simulink subsystem "CF1_SubSystem"  (R2020b)
settings: Solver=VariableStepAuto  StartTime=0.0  StopTime=10.0  RelTol=1e-3
values from neighbouring files (symbols this model uses):
  Hz = HFE    [StateSpaceSimpleObserver.m]
  Ts = 1e-2    (= 0.01)    [balrob_params.m]
undefined symbols (not defined in the file or in its folder): DiscIntNeverNeededParam
settings Model: Creator=umberto  LastModifiedBy=umberto

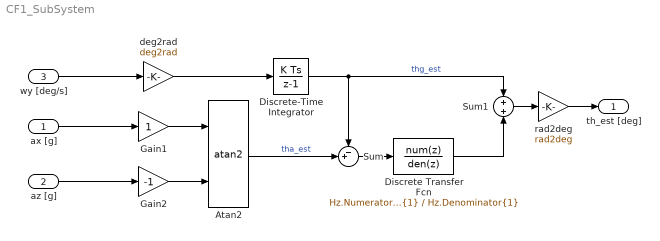
== system CF1_SubSystem ==
  ax [g] : Inport
  az [g] : Inport  Port=2
  wy [deg/s] : Inport  Port=3
  Atan2 : Trigonometry  Operator=atan2
  Discrete Transfer Fcn : DiscreteTransferFcn  Numerator=Hz.Numerator{1}  Denominator=Hz.Denominator{1}  SampleTime=Ts
  Discrete-Time Integrator : DiscreteIntegrator  SampleTime=Ts  ICPrevOutput=DiscIntNeverNeededParam  ICPrevScaledInput=DiscIntNeverNeededParam
  Gain1 : Gain
  Gain2 : Gain  Gain=-1
  Sum : Sum  Inputs=-+|
  Sum1 : Sum
  deg2rad : Gain  Gain=deg2rad
  rad2deg : Gain  Gain=rad2deg
  th_est [deg] : Outport
  wires:
  wy [deg/s]/1 -> deg2rad/1
  deg2rad/1 -> Discrete-Time Integrator/1
  ax [g]/1 -> Gain1/1
  az [g]/1 -> Gain2/1
  Discrete-Time Integrator/1 -> Sum1/1, Sum/1  "thg_est"
  Gain1/1 -> Atan2/1
  Gain2/1 -> Atan2/2
  Atan2/1 -> Sum/2  "tha_est"
  Sum/1 -> Discrete Transfer Fcn/1
  Discrete Transfer Fcn/1 -> Sum1/2
  Sum1/1 -> rad2deg/1
  rad2deg/1 -> th_est [deg]/1
